simulink model "Oving3Oppg3b"  (R2020b)
settings: Solver=VariableStepAuto  StartTime=0.0  StopTime=1000  RelTol=1e-3
values from neighbouring files (symbols this model uses):
  A = 2.34    [Oving3Oppg3Variables.mat]
  C_d = 0.24    [Oving3Oppg3Variables.mat]
  d = 0    [Oving3Oppg3Variables.mat]
  m = 2170    [Oving3Oppg3Variables.mat]
  rho = 1.225    [Oving3Oppg3Variables.mat]
  v_0 = 25    [Oving3Oppg3Variables.mat]
settings Model: Creator=crezl  LastModifiedBy=crezl

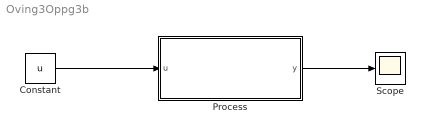
== system Oving3Oppg3b ==
  Constant : Constant  Value=u
  Process : Subsystem
  Scope : Scope
  wires:
  Constant/1 -> Process/1(u)
  Process/1(y) -> Scope/1

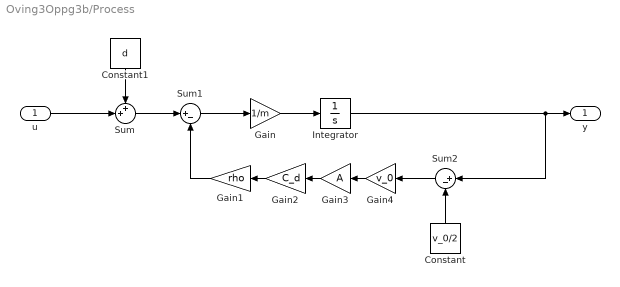
== system Oving3Oppg3b/Process ==
  u : Inport
  Constant : Constant  Value=v_0/2
  Constant1 : Constant  Value=d
  Gain : Gain  Gain=1/m
  Gain1 : Gain  Gain=rho
  Gain2 : Gain  Gain=C_d
  Gain3 : Gain  Gain=A
  Gain4 : Gain  Gain=v_0
  Integrator : Integrator  InitialCondition=1.2*v_0
  Sum : Sum  Inputs=++|
  Sum1 : Sum  Inputs=|+-
  Sum2 : Sum  Inputs=|+-
  y : Outport
  wires:
  Constant1/1 -> Sum/1
  Integrator/1 -> Sum2/1, y/1
  Sum/1 -> Sum1/1
  Gain1/1 -> Sum1/2
  Sum1/1 -> Gain/1
  Gain3/1 -> Gain2/1
  Gain2/1 -> Gain1/1
  Gain/1 -> Integrator/1
  u/1 -> Sum/2
  Gain4/1 -> Gain3/1
  Constant/1 -> Sum2/2
  Sum2/1 -> Gain4/1
